simulink model "model_v4"  (R2023b)
settings: Solver=VariableStepAuto  StartTime=0.0  StopTime=10.0  RelTol=1e-3
(part 1 of 2)
settings Model: Creator=ian20030201  LastModifiedBy=ian20030201

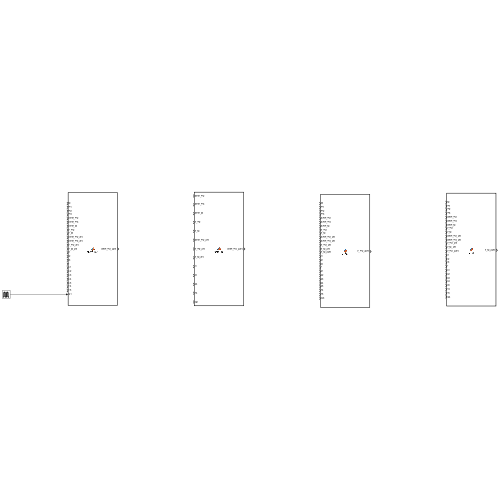
[thumbnail: Simulink's stored preview of the top-level diagram]
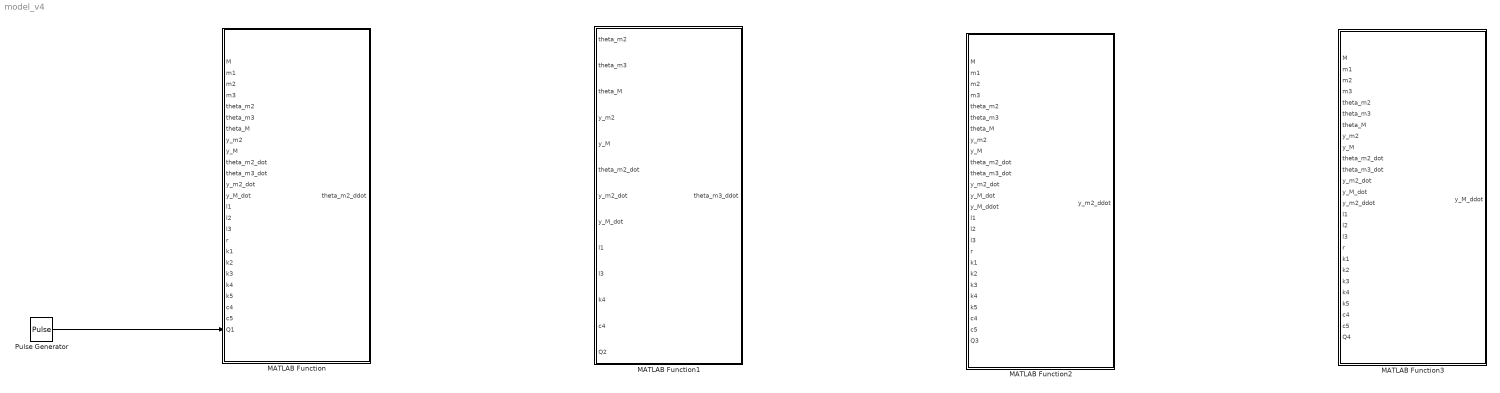
== system model_v4 ==
  MATLAB Function : MATLAB Function  TreatAsAtomicUnit=on
  MATLAB Function1 : MATLAB Function  TreatAsAtomicUnit=on
  MATLAB Function2 : MATLAB Function  TreatAsAtomicUnit=on
  MATLAB Function3 : MATLAB Function  TreatAsAtomicUnit=on
  Pulse Generator : DiscretePulseGenerator  PulseType=Time based  Period=10  PulseWidth=5
  wires:
  Pulse Generator/1 -> MATLAB Function/25(Q1)

== matlab function model_v4/MATLAB Function3 ==
  data: M input; y_M_ddot output; m1 input; m2 input; m3 input; theta_m2 input; theta_m3 input; theta_M input; y_m2 input; y_M input; theta_m2_dot input; theta_m3_dot input; y_m2_dot input; y_M_dot input; y_m2_ddot input; l1 input; l2 input; l3 input; r input; k1 input; k2 input; k3 input; k4 input; k5 input; c4 input; c5 input; Q4 input
function y_M_ddot = y_M(M, m1, m2, m3, theta_m2, theta_m3, theta_M, y_m2, y_M, theta_m2_dot, theta_m3_dot, y_m2_dot, y_M_dot, y_m2_ddot, l1, l2, l3, r, k1, k2, k3, k4, k5, c4, c5, Q4)

g = 9.81;
y_M_ddot = (-M*g*sqrt((l3*sin(theta_m3) - y_M*tan(theta_M) + y_m2*tan(theta_M))^2 + (l1*theta_m2 + l3*cos(theta_m3) - y_M - y_m2)^2)*(l3*sin(theta_m3) - y_M*tan(theta_M) + y_m2*tan(theta_M))^2*cos(theta_M)*tan(theta_M) - M*g*sqrt((l3*sin(theta_m3) - y_M*tan(theta_M) + y_m2*tan(theta_M))^2 + (l1*theta_m2 + l3*cos(theta_m3) - y_M - y_m2)^2)*(l1*theta_m2 + l3*cos(theta_m3) - y_M - y_m2)^2*cos(theta_M)*tan(theta_M) + Q4*sqrt((l3*sin(theta_m3) - y_M*tan(theta_M) + y_m2*tan(theta_M))^2 + (l1*theta_m2 + l3*cos(theta_m3) - y_M - y_m2)^2)*(l3*sin(theta_m3) - y_M*tan(theta_M) + y_m2*tan(theta_M))^2*tan(theta_M)^2 + Q4*sqrt((l3*sin(theta_m3) - y_M*tan(theta_M) + y_m2*tan(theta_M))^2 + (l1*theta_m2 + l3*cos(theta_m3) - y_M - y_m2)^2)*(l1*theta_m2 + l3*cos(theta_m3) - y_M - y_m2)^2*tan(theta_M)^2 + c4*l1^3*theta_m2^2*theta_m2_dot*sqrt((l3*sin(theta_m3) - y_M*tan(theta_M) + y_m2*tan(theta_M))^2 + (l1*theta_m2 + l3*cos(theta_m3) - y_M - y_m2)^2)*tan(theta_M)^2 - c4*l1^2*l3*theta_m2^2*theta_m3_dot*sqrt((l3*sin(theta_m3) - y_M*tan(theta_M) + y_m2*tan(theta_M))^2 + (l1*theta_m2 + l3*cos(theta_m3) - y_M - y_m2)^2)*sin(theta_m3)*tan(theta_M)^2 + c4*l1^2*l3*theta_m2*theta_m2_dot*sqrt((l3*sin(theta_m3) - y_M*tan(theta_M) + y_m2*tan(theta_M))^2 + (l1*theta_m2 + l3*cos(theta_m3) - y_M - y_m2)^2)*sin(theta_m3)*tan(theta_M)^3 + 2.0*c4*l1^2*l3*theta_m2*theta_m2_dot*sqrt((l3*sin(theta_m3) - y_M*tan(theta_M) + y_m2*tan(theta_M))^2 + (l1*theta_m2 + l3*cos(theta_m3) - y_M - y_m2)^2)*cos(theta_m3)*tan(theta_M)^2 - c4*l1^2*theta_m2^2*y_M_dot*sqrt((l3*sin(theta_m3) - y_M*tan(theta_M) + y_m2*tan(theta_M))^2 + (l1*theta_m2 + l3*cos(theta_m3) - y_M - y_m2)^2)*tan(theta_M)^2 - c4*l1^2*theta_m2^2*y_m2_dot*sqrt((l3*sin(theta_m3) - y_M*tan(theta_M) + y_m2*tan(theta_M))^2 + (l1*theta_m2 + l3*cos(theta_m3) - y_M - y_m2)^2)*tan(theta_M)^2 - c4*l1^2*theta_m2*theta_m2_dot*y_M*sqrt((l3*sin(theta_m3) - y_M*tan(theta_M) + y_m2*tan(theta_M))^2 + (l1*theta_m2 + l3*cos(theta_m3) - y_M - y_m2)^2)*tan(theta_M)^4 - 2.0*c4*l1^2*theta_m2*theta_m2_dot*y_M*sqrt((l3*sin(theta_m3) - y_M*tan(theta_M) + y_m2*tan(theta_M))^2 + (l1*theta_m2 + l3*cos(theta_m3) - y_M - y_m2)^2)*tan(theta_M)^2 + c4*l1^2*theta_m2*theta_m2_dot*y_m2*sqrt((l3*sin(theta_m3) - y_M*tan(theta_M) + y_m2*tan(theta_M))^2 + (l1*theta_m2 + l3*cos(theta_m3) - y_M - y_m2)^2)*tan(theta_M)^4 - 2.0*c4*l1^2*theta_m2*theta_m2_dot*y_m2*sqrt((l3*sin(theta_m3) - y_M*tan(theta_M) + y_m2*tan(theta_M))^2 + (l1*theta_m2 + l3*cos(theta_m3) - y_M - y_m2)^2)*tan(theta_M)^2 - c4*l1*l3^2*theta_m2*theta_m3_dot*sqrt((l3*sin(theta_m3) - y_M*tan(theta_M) + y_m2*tan(theta_M))^2 + (l1*theta_m2 + l3*cos(theta_m3) - y_M - y_m2)^2)*sin(theta_m3)^2*tan(theta_M)^3 - c4*l1*l3^2*theta_m2*theta_m3_dot*sqrt((l3*sin(theta_m3) - y_M*tan(theta_M) + y_m2*tan(theta_M))^2 + (l1*theta_m2 + l3*cos(theta_m3) - y_M - y_m2)^2)*sin(theta_m3)*cos(theta_m3)*tan(theta_M)^2 + c4*l1*l3^2*theta_m2_dot*sqrt((l3*sin(theta_m3) - y_M*tan(theta_M) + y_m2*tan(theta_M))^2 + (l1*theta_m2 + l3*cos(theta_m3) - y_M - y_m2)^2)*sin(theta_m3)*cos(theta_m3)*tan(theta_M)^3 + c4*l1*l3^2*theta_m2_dot*sqrt((l3*sin(theta_m3) - y_M*tan(theta_M) + y_m2*tan(theta_M))^2 + (l1*theta_m2 + l3*cos(theta_m3) - y_M - y_m2)^2)*cos(theta_m3)^2*tan(theta_M)^2 + c4*l1*l3*theta_m2*theta_m3_dot*y_M*sqrt((l3*sin(theta_m3) - y_M*tan(theta_M) + y_m2*tan(theta_M))^2 + (l1*theta_m2 + l3*cos(theta_m3) - y_M - y_m2)^2)*sin(theta_m3)*tan(theta_M)^4 + 2.0*c4*l1*l3*theta_m2*theta_m3_dot*y_M*sqrt((l3*sin(theta_m3) - y_M*tan(theta_M) + y_m2*tan(theta_M))^2 + (l1*theta_m2 + l3*cos(theta_m3) - y_M - y_m2)^2)*sin(theta_m3)*tan(theta_M)^2 - c4*l1*l3*theta_m2*theta_m3_dot*y_M*sqrt((l3*sin(theta_m3) - y_M*tan(theta_M) + y_m2*tan(theta_M))^2 + (l1*theta_m2 + l3*cos(theta_m3) - y_M - y_m2)^2)*cos(theta_m3)*tan(theta_M)^3 - c4*l1*l3*theta_m2*theta_m3_dot*y_m2*sqrt((l3*sin(theta_m3) - y_M*tan(theta_M) + y_m2*tan(theta_M))^2 + (l1*theta_m2 + l3*cos(theta_m3) - y_M - y_m2)^2)*sin(theta_m3)*tan(theta_M)^4 + 2.0*c4*l1*l3*theta_m2*theta_m3_dot*y_m2*sqrt((l3*sin(theta_m3) - y_M*tan(theta_M) + y_m2*tan(theta_M))^2 + (l1*theta_m2 + l3*cos(theta_m3) - y_M - y_m2)^2)*sin(theta_m3)*tan(theta_M)^2 + c4*l1*l3*theta_m2*theta_m3_dot*y_m2*sqrt((l3*sin(theta_m3) - y_M*tan(theta_M) + y_m2*tan(theta_M))^2 + (l1*theta_m2 + l3*cos(theta_m3) - y_M - y_m2)^2)*cos(theta_m3)*tan(theta_M)^3 - 2.0*c4*l1*l3*theta_m2*y_M_dot*sqrt((l3*sin(theta_m3) - y_M*tan(theta_M) + y_m2*tan(theta_M))^2 + (l1*theta_m2 + l3*cos(theta_m3) - y_M - y_m2)^2)*sin(theta_m3)*tan(theta_M)^3 - 2.0*c4*l1*l3*theta_m2*y_M_dot*sqrt((l3*sin(theta_m3) - y_M*tan(theta_M) + y_m2*tan(theta_M))^2 + (l1*theta_m2 + l3*cos(theta_m3) - y_M - y_m2)^2)*cos(theta_m3)*tan(theta_M)^2 - 2.0*c4*l1*l3*theta_m2*y_m2_dot*sqrt((l3*sin(theta_m3) - y_M*tan(theta_M) + y_m2*tan(theta_M))^2 + (l1*theta_m2 + l3*cos(theta_m3) - y_M - y_m2)^2)*cos(theta_m3)*tan(theta_M)^2 - c4*l1*l3*theta_m2_dot*y_M*sqrt((l3*sin(theta_m3) - y_M*tan(theta_M) + y_m2*tan(theta_M))^2 + (l1*theta_m2 + l3*cos(theta_m3) - y_M - y_m2)^2)*sin(theta_m3)*tan(theta_M)^3 - c4*l1*l3*theta_m2_dot*y_M*sqrt((l3*sin(theta_m3) - y_M*tan(theta_M) + y_m2*tan(theta_M))^2 + (l1*theta_m2 + l3*cos(theta_m3) - y_M - y_m2)^2)*cos(theta_m3)*tan(theta_M)^4 - 2.0*c4*l1*l3*theta_m2_dot*y_M*sqrt((l3*sin(theta_m3) - y_M*tan(theta_M) + y_m2*tan(theta_M))^2 + (l1*theta_m2 + l3*cos(theta_m3) - y_M - y_m2)^2)*cos(theta_m3)*tan(theta_M)^2 - c4*l1*l3*theta_m2_dot*y_m2*sqrt((l3*sin(theta_m3) - y_M*tan(theta_M) + y_m2*tan(theta_M))^2 + (l1*theta_m2 + l3*cos(theta_m3) - y_M - y_m2)^2)*sin(theta_m3)*tan(theta_M)^3 + c4*l1*l3*theta_m2_dot*y_m2*sqrt((l3*sin(theta_m3) - y_M*tan(theta_M) + y_m2*tan(theta_M))^2 + (l1*theta_m2 + l3*cos(theta_m3) - y_M - y_m2)^2)*cos(theta_m3)*tan(theta_M)^4 - 2.0*c4*l1*l3*theta_m2_dot*y_m2*sqrt((l3*sin(theta_m3) - y_M*tan(theta_M) + y_m2*tan(theta_M))^2 + (l1*theta_m2 + l3*cos(theta_m3) - y_M - y_m2)^2)*cos(theta_m3)*tan(theta_M)^2 + 2.0*c4*l1*theta_m2*y_M*y_M_dot*sqrt((l3*sin(theta_m3) - y_M*tan(theta_M) + y_m2*tan(theta_M))^2 + (l1*theta_m2 + l3*cos(theta_m3) - y_M - y_m2)^2)*tan(theta_M)^4 + 2.0*c4*l1*theta_m2*y_M*y_M_dot*sqrt((l3*sin(theta_m3) - y_M*tan(theta_M) + y_m2*tan(theta_M))^2 + (l1*theta_m2 + l3*cos(theta_m3) - y_M - y_m2)^2)*tan(theta_M)^2 + 2.0*c4*l1*theta_m2*y_M*y_m2_dot*sqrt((l3*sin(theta_m3) - y_M*tan(theta_M) + y_m2*tan(theta_M))^2 + (l1*theta_m2 + l3*cos(theta_m3) - y_M - y_m2)^2)*tan(theta_M)^2 - 2.0*c4*l1*theta_m2*y_M_dot*y_m2*sqrt((l3*sin(theta_m3) - y_M*tan(theta_M) + y_m2*tan(theta_M))^2 + (l1*theta_m2 + l3*cos(theta_m3) - y_M - y_m2)^2)*tan(theta_M)^4 + 2.0*c4*l1*theta_m2*y_M_dot*y_m2*sqrt((l3*sin(theta_m3) - y_M*tan(theta_M) + y_m2*tan(theta_M))^2 + (l1*theta_m2 + l3*cos(theta_m3) - y_M - y_m2)^2)*tan(theta_M)^2 + 2.0*c4*l1*theta_m2*y_m2*y_m2_dot*sqrt((l3*sin(theta_m3) - y_M*tan(theta_M) + y_m2*tan(theta_M))^2 + (l1*theta_m2 + l3*cos(theta_m3) - y_M - y_m2)^2)*tan(theta_M)^2 + c4*l1*theta_m2_dot*y_M^2*sqrt((l3*sin(theta_m3) - y_M*tan(theta_M) + y_m2*tan(theta_M))^2 + (l1*theta_m2 + l3*cos(theta_m3) - y_M - y_m2)^2)*tan(theta_M)^4 + c4*l1*theta_m2_dot*y_M^2*sqrt((l3*sin(theta_m3) - y_M*tan(theta_M) + y_m2*tan(theta_M))^2 + (l1*theta_m2 + l3*cos(theta_m3) - y_M - y_m2)^2)*tan(theta_M)^2 + 2.0*c4*l1*theta_m2_dot*y_M*y_m2*sqrt((l3*sin(theta_m3) - y_M*tan(theta_M) + y_m2*tan(theta_M))^2 + (l1*theta_m2 + l3*cos(theta_m3) - y_M - y_m2)^2)*tan(theta_M)^2 - c4*l1*theta_m2_dot*y_m2^2*sqrt((l3*sin(theta_m3) - y_M*tan(theta_M) + y_m2*tan(theta_M))^2 + (l1*theta_m2 + l3*cos(theta_m3) - y_M - y_m2)^2)*tan(theta_M)^4 + c4*l1*theta_m2_dot*y_m2^2*sqrt((l3*sin(theta_m3) - y_M*tan(theta_M) + y_m2*tan(theta_M))^2 + (l1*theta_m2 + l3*cos(theta_m3) - y_M - y_m2)^2)*tan(theta_M)^2 + c4*l3^2*theta_m3_dot*y_M*sqrt((l3*sin(theta_m3) - y_M*tan(theta_M) + y_m2*tan(theta_M))^2 + (l1*theta_m2 + l3*cos(theta_m3) - y_M - y_m2)^2)*sin(theta_m3)^2*tan(theta_M)^3 - c4*l3^2*theta_m3_dot*y_M*sqrt((l3*sin(theta_m3) - y_M*tan(theta_M) + y_m2*tan(theta_M))^2 + (l1*theta_m2 + l3*cos(theta_m3) - y_M - y_m2)^2)*sin(theta_m3)*cos(theta_m3)*tan(theta_M)^4 + c4*l3^2*theta_m3_dot*y_M*sqrt((l3*sin(theta_m3) - y_M*tan(theta_M) + y_m2*tan(theta_M))^2 + (l1*theta_m2 + l3*cos(theta_m3) - y_M - y_m2)^2)*sin(theta_m3)*cos(theta_m3)*tan(theta_M)^2 - c4*l3^2*theta_m3_dot*y_M*sqrt((l3*sin(theta_m3) - y_M*tan(theta_M) + y_m2*tan(theta_M))^2 + (l1*theta_m2 + l3*cos(theta_m3) - y_M - y_m2)^2)*cos(theta_m3)^2*tan(theta_M)^3 + c4*l3^2*theta_m3_dot*y_m2*sqrt((l3*sin(theta_m3) - y_M*tan(theta_M) + y_m2*tan(theta_M))^2 + (l1*theta_m2 + l3*cos(theta_m3) - y_M - y_m2)^2)*sin(theta_m3)^2*tan(theta_M)^3 + c4*l3^2*theta_m3_dot*y_m2*sqrt((l3*sin(theta_m3) - y_M*tan(theta_M) + y_m2*tan(theta_M))^2 + (l1*theta_m2 + l3*cos(theta_m3) - y_M - y_m2)^2)*sin(theta_m3)*cos(theta_m3)*tan(theta_M)^4 + c4*l3^2*theta_m3_dot*y_m2*sqrt((l3*sin(theta_m3) - y_M*tan(theta_M) + y_m2*tan(theta_M))^2 + (l1*theta_m2 + l3*cos(theta_m3) - y_M - y_m2)^2)*sin(theta_m3)*cos(theta_m3)*tan(theta_M)^2 + c4*l3^2*theta_m3_dot*y_m2*sqrt((l3*sin(theta_m3) - y_M*tan(theta_M) + y_m2*tan(theta_M))^2 + (l1*theta_m2 + l3*cos(theta_m3) - y_M - y_m2)^2)*cos(theta_m3)^2*tan(theta_M)^3 - c4*l3^2*y_M_dot*sqrt((l3*sin(theta_m3) - y_M*tan(theta_M) + y_m2*tan(theta_M))^2 + (l1*theta_m2 + l3*cos(theta_m3) - y_M - y_m2)^2)*sin(theta_m3)^2*tan(theta_M)^4 - 2.0*c4*l3^2*y_M_dot*sqrt((l3*sin(theta_m3) - y_M*tan(theta_M) + y_m2*tan(theta_M))^2 + (l1*theta_m2 + l3*cos(theta_m3) - y_M - y_m2)^2)*sin(theta_m3)*cos(theta_m3)*tan(theta_M)^3 - c4*l3^2*y_M_dot*sqrt((l3*sin(theta_m3) - y_M*tan(theta_M) + y_m2*tan(theta_M))^2 + (l1*theta_m2 + l3*cos(theta_m3) - y_M - y_m2)^2)*cos(theta_m3)^2*tan(theta_M)^2 + c4*l3^2*y_m2_dot*sqrt((l3*sin(theta_m3) - y_M*tan(theta_M) + y_m2*tan(theta_M))^2 + (l1*theta_m2 + l3*cos(theta_m3) - y_M - y_m2)^2)*sin(theta_m3)^2*tan(theta_M)^4 - c4*l3^2*y_m2_dot*sqrt((l3*sin(theta_m3) - y_M*tan(theta_M) + y_m2*tan(theta_M))^2 + (l1*theta_m2 + l3*cos(theta_m3) - y_M - y_m2)^2)*cos(theta_m3)^2*tan(theta_M)^2 - c4*l3*theta_m3_dot*y_M^2*sqrt((l3*sin(theta_m3) - y_M*tan(theta_M) + y_m2*tan(theta_M))^2 + (l1*theta_m2 + l3*cos(theta_m3) - y_M - y_m2)^2)*sin(theta_m3)*tan(theta_M)^4 - c4*l3*theta_m3_dot*y_M^2*sqrt((l3*sin(theta_m3) - y_M*tan(theta_M) + y_m2*tan(theta_M))^2 + (l1*theta_m2 + l3*cos(theta_m3) - y_M - y_m2)^2)*sin(theta_m3)*tan(theta_M)^2 + c4*l3*theta_m3_dot*y_M^2*sqrt((l3*sin(theta_m3) - y_M*tan(theta_M) + y_m2*tan(theta_M))^2 + (l1*theta_m2 + l3*cos(theta_m3) - y_M - y_m2)^2)*cos(theta_m3)*tan(theta_M)^5 + c4*l3*theta_m3_dot*y_M^2*sqrt((l3*sin(theta_m3) - y_M*tan(theta_M) + y_m2*tan(theta_M))^2 + (l1*theta_m2 + l3*cos(theta_m3) - y_M - y_m2)^2)*cos(theta_m3)*tan(theta_M)^3 - 2.0*c4*l3*theta_m3_dot*y_M*y_m2*sqrt((l3*sin(theta_m3) - y_M*tan(theta_M) + y_m2*tan(theta_M))^2 + (l1*theta_m2 + l3*cos(theta_m3) - y_M - y_m2)^2)*sin(theta_m3)*tan(theta_M)^2 - 2.0*c4*l3*theta_m3_dot*y_M*y_m2*sqrt((l3*sin(theta_m3) - y_M*tan(theta_M) + y_m2*tan(theta_M))^2 + (l1*theta_m2 + l3*cos(theta_m3) - y_M - y_m2)^2)*cos(theta_m3)*tan(theta_M)^5 + c4*l3*theta_m3_dot*y_m2^2*sqrt((l3*sin(theta_m3) - y_M*tan(theta_M) + y_m2*tan(theta_M))^2 + (l1*theta_m2 + l3*cos(theta_m3) - y_M - y_m2)^2)*sin(theta_m3)*tan(theta_M)^4 - c4*l3*theta_m3_dot*y_m2^2*sqrt((l3*sin(theta_m3) - y_M*tan(theta_M) + y_m2*tan(theta_M))^2 + (l1*theta_m2 + l3*cos(theta_m3) - y_M - y_m2)^2)*sin(theta_m3)*tan(theta_M)^2 + c4*l3*theta_m3_dot*y_m2^2*sqrt((l3*sin(theta_m3) - y_M*tan(theta_M) + y_m2*tan(theta_M))^2 + (l1*theta_m2 + l3*cos(theta_m3) - y_M - y_m2)^2)*cos(theta_m3)*tan(theta_M)^5 - c4*l3*theta_m3_dot*y_m2^2*sqrt((l3*sin(theta_m3) - y_M*tan(theta_M) + y_m2*tan(theta_M))^2 + (l1*theta_m2 + l3*cos(theta_m3) - y_M - y_m2)^2)*cos(theta_m3)*tan(theta_M)^3 + 2.0*c4*l3*y_M*y_M_dot*sqrt((l3*sin(theta_m3) - y_M*tan(theta_M) + y_m2*tan(theta_M))^2 + (l1*theta_m2 + l3*cos(theta_m3) - y_M - y_m2)^2)*sin(theta_m3)*tan(theta_M)^5 + 2.0*c4*l3*y_M*y_M_dot*sqrt((l3*sin(theta_m3) - y_M*tan(theta_M) + y_m2*tan(theta_M))^2 + (l1*theta_m2 + l3*cos(theta_m3) - y_M - y_m2)^2)*sin(theta_m3)*tan(theta_M)^3 + 2.0*c4*l3*y_M*y_M_dot*sqrt((l3*sin(theta_m3) - y_M*tan(theta_M) + y_m2*tan(theta_M))^2 + (l1*theta_m2 + l3*cos(theta_m3) - y_M - y_m2)^2)*cos(theta_m3)*tan(theta_M)^4 + 2.0*c4*l3*y_M*y_M_dot*sqrt((l3*sin(theta_m3) - y_M*tan(theta_M) + y_m2*tan(theta_M))^2 + (l1*theta_m2 + l3*cos(theta_m3) - y_M - y_m2)^2)*cos(theta_m3)*tan(theta_M)^2 - 2.0*c4*l3*y_M*y_m2_dot*sqrt((l3*sin(theta_m3) - y_M*tan(theta_M) + y_m2*tan(theta_M))^2 + (l1*theta_m2 + l3*cos(theta_m3) - y_M - y_m2)^2)*sin(theta_m3)*tan(theta_M)^5 + 2.0*c4*l3*y_M*y_m2_dot*sqrt((l3*sin(theta_m3) - y_M*tan(theta_M) + y_m2*tan(theta_M))^2 + (l1*theta_m2 + l3*cos(theta_m3) - y_M - y_m2)^2)*cos(theta_m3)*tan(theta_M)^2 - 2.0*c4*l3*y_M_dot*y_m2*sqrt((l3*sin(theta_m3) - y_M*tan(theta_M) + y_m2*tan(theta_M))^2 + (l1*theta_m2 + l3*cos(theta_m3) - y_M - y_m2)^2)*sin(theta_m3)*tan(theta_M)^5 + 2.0*c4*l3*y_M_dot*y_m2*sqrt((l3*sin(theta_m3) - y_M*tan(theta_M) + y_m2*tan(theta_M))^2 + (l1*theta_m2 + l3*cos(theta_m3) - y_M - y_m2)^2)*sin(theta_m3)*tan(theta_M)^3 - 2.0*c4*l3*y_M_dot*y_m2*sqrt((l3*sin(theta_m3) - y_M*tan(theta_M) + y_m2*tan(theta_M))^2 + (l1*theta_m2 + l3*cos(theta_m3) - y_M - y_m2)^2)*cos(theta_m3)*tan(theta_M)^4 + 2.0*c4*l3*y_M_dot*y_m2*sqrt((l3*sin(theta_m3) - y_M*tan(theta_M) + y_m2*tan(theta_M))^2 + (l1*theta_m2 + l3*cos(theta_m3) - y_M - y_m2)^2)*cos(theta_m3)*tan(theta_M)^2 + 2.0*c4*l3*y_m2*y_m2_dot*sqrt((l3*sin(theta_m3) - y_M*tan(theta_M) + y_m2*tan(theta_M))^2 + (l1*theta_m2 + l3*cos(theta_m3) - y_M - y_m2)^2)*sin(theta_m3)*tan(theta_M)^5 + 2.0*c4*l3*y_m2*y_m2_dot*sqrt((l3*sin(theta_m3) - y_M*tan(theta_M) + y_m2*tan(theta_M))^2 + (l1*theta_m2 + l3*cos(theta_m3) - y_M - y_m2)^2)*cos(theta_m3)*tan(theta_M)^2 - c4*y_M^2*y_M_dot*sqrt((l3*sin(theta_m3) - y_M*tan(theta_M) + y_m2*tan(theta_M))^2 + (l1*theta_m2 + l3*cos(theta_m3) - y_M - y_m2)^2)*tan(theta_M)^6 - 2.0*c4*y_M^2*y_M_dot*sqrt((l3*sin(theta_m3) - y_M*tan(theta_M) + y_m2*tan(theta_M))^2 + (l1*theta_m2 + l3*cos(theta_m3) - y_M - y_m2)^2)*tan(theta_M)^4 - c4*y_M^2*y_M_dot*sqrt((l3*sin(theta_m3) - y_M*tan(theta_M) + y_m2*tan(theta_M))^2 + (l1*theta_m2 + l3*cos(theta_m3) - y_M - y_m2)^2)*tan(theta_M)^2 + c4*y_M^2*y_m2_dot*sqrt((l3*sin(theta_m3) - y_M*tan(theta_M) + y_m2*tan(theta_M))^2 + (l1*theta_m2 + l3*cos(theta_m3) - y_M - y_m2)^2)*tan(theta_M)^6 - c4*y_M^2*y_m2_dot*sqrt((l3*sin(theta_m3) - y_M*tan(theta_M) + y_m2*tan(theta_M))^2 + (l1*theta_m2 + l3*cos(theta_m3) - y_M - y_m2)^2)*tan(theta_M)^2 + 2.0*c4*y_M*y_M_dot*y_m2*sqrt((l3*sin(theta_m3) - y_M*tan(theta_M) + y_m2*tan(theta_M))^2 + (l1*theta_m2 + l3*cos(theta_m3) - y_M - y_m2)^2)*tan(theta_M)^6 - 2.0*c4*y_M*y_M_dot*y_m2*sqrt((l3*sin(theta_m3) - y_M*tan(theta_M) + y_m2*tan(theta_M))^2 + (l1*theta_m2 + l3*cos(theta_m3) - y_M - y_m2)^2)*tan(theta_M)^2 - 2.0*c4*y_M*y_m2*y_m2_dot*sqrt((l3*sin(theta_m3) - y_M*tan(theta_M) + y_m2*tan(theta_M))^2 + (l1*theta_m2 + l3*cos(theta_m3) - y_M - y_m2)^2)*tan(theta_M)^6 - 2.0*c4*y_M*y_m2*y_m2_dot*sqrt((l3*sin(theta_m3) - y_M*tan(theta_M) + y_m2*tan(theta_M))^2 + (l1*theta_m2 + l3*cos(theta_m3) - y_M - y_m2)^2)*tan(theta_M)^2 - c4*y_M_dot*y_m2^2*sqrt((l3*sin(theta_m3) - y_M*tan(theta_M) + y_m2*tan(theta_M))^2 + (l1*theta_m2 + l3*cos(theta_m3) - y_M - y_m2)^2)*tan(theta_M)^6 + 2.0*c4*y_M_dot*y_m2^2*sqrt((l3*sin(theta_m3) - y_M*tan(theta_M) + y_m2*tan(theta_M))^2 + (l1*theta_m2 + l3*cos(theta_m3) - y_M - y_m2)^2)*tan(theta_M)^4 - c4*y_M_dot*y_m2^2*sqrt((l3*sin(theta_m3) - y_M*tan(theta_M) + y_m2*tan(theta_M))^2 + (l1*theta_m2 + l3*cos(theta_m3) - y_M - y_m2)^2)*tan(theta_M)^2 + c4*y_m2^2*y_m2_dot*sqrt((l3*sin(theta_m3) - y_M*tan(theta_M) + y_m2*tan(theta_M))^2 + (l1*theta_m2 + l3*cos(theta_m3) - y_M - y_m2)^2)*tan(theta_M)^6 - c4*y_m2^2*y_m2_dot*sqrt((l3*sin(theta_m3) - y_M*tan(theta_M) + y_m2*tan(theta_M))^2 + (l1*theta_m2 + l3*cos(theta_m3) - y_M - y_m2)^2)*tan(theta_M)^2 - c5*y_M_dot*sqrt((l3*sin(theta_m3) - y_M*tan(theta_M) + y_m2*tan(theta_M))^2 + (l1*theta_m2 + l3*cos(theta_m3) - y_M - y_m2)^2)*(l3*sin(theta_m3) - y_M*tan(theta_M) + y_m2*tan(theta_M))^2 - c5*y_M_dot*sqrt((l3*sin(theta_m3) - y_M*tan(theta_M) + y_m2*tan(theta_M))^2 + (l1*theta_m2 + l3*cos(theta_m3) - y_M - y_m2)^2)*(l1*theta_m2 + l3*cos(theta_m3) - y_M - y_m2)^2 + c5*y_m2_dot*sqrt((l3*sin(theta_m3) - y_M*tan(theta_M) + y_m2*tan(theta_M))^2 + (l1*theta_m2 + l3*cos(theta_m3) - y_M - y_m2)^2)*(l3*sin(theta_m3) - y_M*tan(theta_M) + y_m2*tan(theta_M))^2 + c5*y_m2_dot*sqrt((l3*sin(theta_m3) - y_M*tan(theta_M) + y_m2*tan(theta_M))^2 + (l1*theta_m2 + l3*cos(theta_m3) - y_M - y_m2)^2)*(l1*theta_m2 + l3*cos(theta_m3) - y_M - y_m2)^2 - k4*l1*l3*theta_m2*(l3*sin(theta_m3) - y_M*tan(theta_M) + y_m2*tan(theta_M))^2*tan(theta_M)^2 - k4*l1*l3*theta_m2*(l1*theta_m2 + l3*cos(theta_m3) - y_M - y_m2)^2*tan(theta_M)^2 + k4*l1*theta_m2*sqrt((l3*sin(theta_m3) - y_M*tan(theta_M) + y_m2*tan(theta_M))^2 + (l1*theta_m2 + l3*cos(theta_m3) - y_M - y_m2)^2)*(l3*sin(theta_m3) - y_M*tan(theta_M) + y_m2*tan(theta_M))^2*tan(theta_M)^2 + k4*l1*theta_m2*sqrt((l3*sin(theta_m3) - y_M*tan(theta_M) + y_m2*tan(theta_M))^2 + (l1*theta_m2 + l3*cos(theta_m3) - y_M - y_m2)^2)*(l1*theta_m2 + l3*cos(theta_m3) - y_M - y_m2)^2*tan(theta_M)^2 - k4*l3^2*(l3*sin(theta_m3) - y_M*tan(theta_M) + y_m2*tan(theta_M))^2*sin(theta_m3)*tan(theta_M)^3 - k4*l3^2*(l3*sin(theta_m3) - y_M*tan(theta_M) + y_m2*tan(theta_M))^2*cos(theta_m3)*tan(theta_M)^2 - k4*l3^2*(l1*theta_m2 + l3*cos(theta_m3) - y_M - y_m2)^2*sin(theta_m3)*tan(theta_M)^3 - k4*l3^2*(l1*theta_m2 + l3*cos(theta_m3) - y_M - y_m2)^2*cos(theta_m3)*tan(theta_M)^2 + k4*l3*y_M*(l3*sin(theta_m3) - y_M*tan(theta_M) + y_m2*tan(theta_M))^2*tan(theta_M)^4 + k4*l3*y_M*(l3*sin(theta_m3) - y_M*tan(theta_M) + y_m2*tan(theta_M))^2*tan(theta_M)^2 + k4*l3*y_M*(l1*theta_m2 + l3*cos(theta_m3) - y_M - y_m2)^2*tan(theta_M)^4 + k4*l3*y_M*(l1*theta_m2 + l3*cos(theta_m3) - y_M - y_m2)^2*tan(theta_M)^2 - k4*l3*y_m2*(l3*sin(theta_m3) - y_M*tan(theta_M) + y_m2*tan(theta_M))^2*tan(theta_M)^4 + k4*l3*y_m2*(l3*sin(theta_m3) - y_M*tan(theta_M) + y_m2*tan(theta_M))^2*tan(theta_M)^2 - k4*l3*y_m2*(l1*theta_m2 + l3*cos(theta_m3) - y_M - y_m2)^2*tan(theta_M)^4 + k4*l3*y_m2*(l1*theta_m2 + l3*cos(theta_m3) - y_M - y_m2)^2*tan(theta_M)^2 + k4*l3*sqrt((l3*sin(theta_m3) - y_M*tan(theta_M) + y_m2*tan(theta_M))^2 + (l1*theta_m2 + l3*cos(theta_m3) - y_M - y_m2)^2)*(l3*sin(theta_m3) - y_M*tan(theta_M) + y_m2*tan(theta_M))^2*sin(theta_m3)*tan(theta_M)^3 + k4*l3*sqrt((l3*sin(theta_m3) - y_M*tan(theta_M) + y_m2*tan(theta_M))^2 + (l1*theta_m2 + l3*cos(theta_m3) - y_M - y_m2)^2)*(l3*sin(theta_m3) - y_M*tan(theta_M) + y_m2*tan(theta_M))^2*cos(theta_m3)*tan(theta_M)^2 + k4*l3*sqrt((l3*sin(theta_m3) - y_M*tan(theta_M) + y_m2*tan(theta_M))^2 + (l1*theta_m2 + l3*cos(theta_m3) - y_M - y_m2)^2)*(l1*theta_m2 + l3*cos(theta_m3) - y_M - y_m2)^2*sin(theta_m3)*tan(theta_M)^3 + k4*l3*sqrt((l3*sin(theta_m3) - y_M*tan(theta_M) + y_m2*tan(theta_M))^2 + (l1*theta_m2 + l3*cos(theta_m3) - y_M - y_m2)^2)*(l1*theta_m2 + l3*cos(theta_m3) - y_M - y_m2)^2*cos(theta_m3)*tan(theta_M)^2 - k4*y_M*sqrt((l3*sin(theta_m3) - y_M*tan(theta_M) + y_m2*tan(theta_M))^2 + (l1*theta_m2 + l3*cos(theta_m3) - y_M - y_m2)^2)*(l3*sin(theta_m3) - y_M*tan(theta_M) + y_m2*tan(theta_M))^2*tan(theta_M)^4 - k4*y_M*sqrt((l3*sin(theta_m3) - y_M*tan(theta_M) + y_m2*tan(theta_M))^2 + (l1*theta_m2 + l3*cos(theta_m3) - y_M - y_m2)^2)*(l3*sin(theta_m3) - y_M*tan(theta_M) + y_m2*tan(theta_M))^2*tan(theta_M)^2 - k4*y_M*sqrt((l3*sin(theta_m3) - y_M*tan(theta_M) + y_m2*tan(theta_M))^2 + (l1*theta_m2 + l3*cos(theta_m3) - y_M - y_m2)^2)*(l1*theta_m2 + l3*cos(theta_m3) - y_M - y_m2)^2*tan(theta_M)^4 - k4*y_M*sqrt((l3*sin(theta_m3) - y_M*tan(theta_M) + y_m2*tan(theta_M))^2 + (l1*theta_m2 + l3*cos(theta_m3) - y_M - y_m2)^2)*(l1*theta_m2 + l3*cos(theta_m3) - y_M - y_m2)^2*tan(theta_M)^2 + k4*y_m2*sqrt((l3*sin(theta_m3) - y_M*tan(theta_M) + y_m2*tan(theta_M))^2 + (l1*theta_m2 + l3*cos(theta_m3) - y_M - y_m2)^2)*(l3*sin(theta_m3) - y_M*tan(theta_M) + y_m2*tan(theta_M))^2*tan(theta_M)^4 - k4*y_m2*sqrt((l3*sin(theta_m3) - y_M*tan(theta_M) + y_m2*tan(theta_M))^2 + (l1*theta_m2 + l3*cos(theta_m3) - y_M - y_m2)^2)*(l3*sin(theta_m3) - y_M*tan(theta_M) + y_m2*tan(theta_M))^2*tan(theta_M)^2 + k4*y_m2*sqrt((l3*sin(theta_m3) - y_M*tan(theta_M) + y_m2*tan(theta_M))^2 + (l1*theta_m2 + l3*cos(theta_m3) - y_M - y_m2)^2)*(l1*theta_m2 + l3*cos(theta_m3) - y_M - y_m2)^2*tan(theta_M)^4 - k4*y_m2*sqrt((l3*sin(theta_m3) - y_M*tan(theta_M) + y_m2*tan(theta_M))^2 + (l1*theta_m2 + l3*cos(theta_m3) - y_M - y_m2)^2)*(l1*theta_m2 + l3*cos(theta_m3) - y_M - y_m2)^2*tan(theta_M)^2 - k5*y_M*sqrt((l3*sin(theta_m3) - y_M*tan(theta_M) + y_m2*tan(theta_M))^2 + (l1*theta_m2 + l3*cos(theta_m3) - y_M - y_m2)^2)*(l3*sin(theta_m3) - y_M*tan(theta_M) + y_m2*tan(theta_M))^2 - k5*y_M*sqrt((l3*sin(theta_m3) - y_M*tan(theta_M) + y_m2*tan(theta_M))^2 + (l1*theta_m2 + l3*cos(theta_m3) - y_M - y_m2)^2)*(l1*theta_m2 + l3*cos(theta_m3) - y_M - y_m2)^2 + k5*y_m2*sqrt((l3*sin(theta_m3) - y_M*tan(theta_M) + y_m2*tan(theta_M))^2 + (l1*theta_m2 + l3*cos(theta_m3) - y_M - y_m2)^2)*(l3*sin(theta_m3) - y_M*tan(theta_M) + y_m2*tan(theta_M))^2 + k5*y_m2*sqrt((l3*sin(theta_m3) - y_M*tan(theta_M) + y_m2*tan(theta_M))^2 + (l1*theta_m2 + l3*cos(theta_m3) - y_M - y_m2)^2)*(l1*theta_m2 + l3*cos(theta_m3) - y_M - y_m2)^2 + m1*y_m2_ddot*sqrt((l3*sin(theta_m3) - y_M*tan(theta_M) + y_m2*tan(theta_M))^2 + (l1*theta_m2 + l3*cos(theta_m3) - y_M - y_m2)^2)*(l3*sin(theta_m3) - y_M*tan(theta_M) + y_m2*tan(theta_M))^2*tan(theta_M)^4 + m1*y_m2_ddot*sqrt((l3*sin(theta_m3) - y_M*tan(theta_M) + y_m2*tan(theta_M))^2 + (l1*theta_m2 + l3*cos(theta_m3) - y_M - y_m2)^2)*(l1*theta_m2 + l3*cos(theta_m3) - y_M - y_m2)^2*tan(theta_M)^4 + m2*y_m2_ddot*sqrt((l3*sin(theta_m3) - y_M*tan(theta_M) + y_m2*tan(theta_M))^2 + (l1*theta_m2 + l3*cos(theta_m3) - y_M - y_m2)^2)*(l3*sin(theta_m3) - y_M*tan(theta_M) + y_m2*tan(theta_M))^2*tan(theta_M)^4 + m2*y_m2_ddot*sqrt((l3*sin(theta_m3) - y_M*tan(theta_M) + y_m2*tan(theta_M))^2 + (l1*theta_m2 + l3*cos(theta_m3) - y_M - y_m2)^2)*(l1*theta_m2 + l3*cos(theta_m3) - y_M - y_m2)^2*tan(theta_M)^4 + m3*y_m2_ddot*sqrt((l3*sin(theta_m3) - y_M*tan(theta_M) + y_m2*tan(theta_M))^2 + (l1*theta_m2 + l3*cos(theta_m3) - y_M - y_m2)^2)*(l3*sin(theta_m3) - y_M*tan(theta_M) + y_m2*tan(theta_M))^2*tan(theta_M)^4 + m3*y_m2_ddot*sqrt((l3*sin(theta_m3) - y_M*tan(theta_M) + y_m2*tan(theta_M))^2 + (l1*theta_m2 + l3*cos(theta_m3) - y_M - y_m2)^2)*(l1*theta_m2 + l3*cos(theta_m3) - y_M - y_m2)^2*tan(theta_M)^4)/(sqrt((l3*sin(theta_m3) - y_M*tan(theta_M) + y_m2*tan(theta_M))^2 + (l1*theta_m2 + l3*cos(theta_m3) - y_M - y_m2)^2)*(M*(l3*sin(theta_m3) - y_M*tan(theta_M) + y_m2*tan(theta_M))^2 + M*(l1*theta_m2 + l3*cos(theta_m3) - y_M - y_m2)^2 + m1*(l3*sin(theta_m3) - y_M*tan(theta_M) + y_m2*tan(theta_M))^2*tan(theta_M)^2 + m1*(l1*theta_m2 + l3*cos(theta_m3) - y_M - y_m2)^2*tan(theta_M)^2 + m2*(l3*sin(theta_m3) - y_M*tan(theta_M) + y_m2*tan(theta_M))^2*tan(theta_M)^2 + m2*(l1*theta_m2 + l3*cos(theta_m3) - y_M - y_m2)^2*tan(theta_M)^2 + m3*(l3*sin(theta_m3) - y_M*tan(theta_M) + y_m2*tan(theta_M))^2*tan(theta_M)^2 + m3*(l1*theta_m2 + l3*cos(theta_m3) - y_M - y_m2)^2*tan(theta_M)^2)*tan(theta_M)^2);

== matlab function model_v4/MATLAB Function1 ==
  data: theta_m2 input; theta_m3 input; theta_M input; y_m2 input; y_M input; theta_m2_dot input; y_m2_dot input; y_M_dot input; l1 input; l3 input; k4 input; c4 input; Q2 input; theta_m3_ddot output
function theta_m3_ddot = theta_m3(theta_m2, theta_m3, theta_M, y_m2, y_M, theta_m2_dot, y_m2_dot, y_M_dot, l1, l3, k4, c4, Q2)

theta_m3_ddot = (-c4*l3*sqrt((l3*sin(theta_m3) - y_M*tan(theta_M) + y_m2*tan(theta_M))^2 + (l1*theta_m2 + l3*cos(theta_m3) - y_M - y_m2)^2)*(-l1^3*theta_m2^2*theta_m2_dot*sin(theta_m3) - 0.5*l1^2*l3*theta_m2*theta_m2_dot*sin(2.0*theta_m3) + l1^2*theta_m2^2*y_M_dot*sin(theta_m3) + l1^2*theta_m2^2*y_m2_dot*sin(theta_m3) + 2.0*l1^2*theta_m2*theta_m2_dot*y_M*sin(theta_m3) - l1^2*theta_m2*theta_m2_dot*y_M*cos(theta_m3)*tan(theta_M) + 2.0*l1^2*theta_m2*theta_m2_dot*y_m2*sin(theta_m3) + l1^2*theta_m2*theta_m2_dot*y_m2*cos(theta_m3)*tan(theta_M) + 0.5*l1*l3*theta_m2*y_M_dot*sin(2.0*theta_m3) - 0.5*l1*l3*theta_m2*y_M_dot*cos(2.0*theta_m3)*tan(theta_M) + 0.5*l1*l3*theta_m2*y_M_dot*tan(theta_M) + 0.5*l1*l3*theta_m2*y_m2_dot*sin(2.0*theta_m3) + 0.5*l1*l3*theta_m2*y_m2_dot*cos(2.0*theta_m3)*tan(theta_M) - 0.5*l1*l3*theta_m2*y_m2_dot*tan(theta_M) + 0.5*l1*l3*theta_m2_dot*y_M*sin(2.0*theta_m3) - 0.5*l1*l3*theta_m2_dot*y_M*cos(2.0*theta_m3)*tan(theta_M) - 0.5*l1*l3*theta_m2_dot*y_M*tan(theta_M) + 0.5*l1*l3*theta_m2_dot*y_m2*sin(2.0*theta_m3) + 0.5*l1*l3*theta_m2_dot*y_m2*cos(2.0*theta_m3)*tan(theta_M) + 0.5*l1*l3*theta_m2_dot*y_m2*tan(theta_M) - l1*theta_m2*y_M*y_M_dot*sin(theta_m3)*tan(theta_M)^2 - 2.0*l1*theta_m2*y_M*y_M_dot*sin(theta_m3) + l1*theta_m2*y_M*y_M_dot*cos(theta_m3)*tan(theta_M) + l1*theta_m2*y_M*y_m2_dot*sin(theta_m3)*tan(theta_M)^2 - 2.0*l1*theta_m2*y_M*y_m2_dot*sin(theta_m3) + l1*theta_m2*y_M*y_m2_dot*cos(theta_m3)*tan(theta_M) + l1*theta_m2*y_M_dot*y_m2*sin(theta_m3)*tan(theta_M)^2 - 2.0*l1*theta_m2*y_M_dot*y_m2*sin(theta_m3) - l1*theta_m2*y_M_dot*y_m2*cos(theta_m3)*tan(theta_M) - l1*theta_m2*y_m2*y_m2_dot*sin(theta_m3)*tan(theta_M)^2 - 2.0*l1*theta_m2*y_m2*y_m2_dot*sin(theta_m3) - l1*theta_m2*y_m2*y_m2_dot*cos(theta_m3)*tan(theta_M) - l1*theta_m2_dot*y_M^2*sin(theta_m3) + l1*theta_m2_dot*y_M^2*cos(theta_m3)*tan(theta_M) - 2.0*l1*theta_m2_dot*y_M*y_m2*sin(theta_m3) - l1*theta_m2_dot*y_m2^2*sin(theta_m3) - l1*theta_m2_dot*y_m2^2*cos(theta_m3)*tan(theta_M) + 0.5*l3*y_M*y_M_dot*sin(2.0*theta_m3)*tan(theta_M)^2 - 0.5*l3*y_M*y_M_dot*sin(2.0*theta_m3) + l3*y_M*y_M_dot*cos(2.0*theta_m3)*tan(theta_M) - 0.5*l3*y_M*y_m2_dot*sin(2.0*theta_m3)*tan(theta_M)^2 - 0.5*l3*y_M*y_m2_dot*sin(2.0*theta_m3) + l3*y_M*y_m2_dot*tan(theta_M) - 0.5*l3*y_M_dot*y_m2*sin(2.0*theta_m3)*tan(theta_M)^2 - 0.5*l3*y_M_dot*y_m2*sin(2.0*theta_m3) - l3*y_M_dot*y_m2*tan(theta_M) + 0.5*l3*y_m2*y_m2_dot*sin(2.0*theta_m3)*tan(theta_M)^2 - 0.5*l3*y_m2*y_m2_dot*sin(2.0*theta_m3) - l3*y_m2*y_m2_dot*cos(2.0*theta_m3)*tan(theta_M) + y_M^2*y_M_dot*sin(theta_m3)*tan(theta_M)^2 + y_M^2*y_M_dot*sin(theta_m3) - y_M^2*y_M_dot*cos(theta_m3)*tan(theta_M)^3 - y_M^2*y_M_dot*cos(theta_m3)*tan(theta_M) - y_M^2*y_m2_dot*sin(theta_m3)*tan(theta_M)^2 + y_M^2*y_m2_dot*sin(theta_m3) + y_M^2*y_m2_dot*cos(theta_m3)*tan(theta_M)^3 - y_M^2*y_m2_dot*cos(theta_m3)*tan(theta_M) + 2.0*y_M*y_M_dot*y_m2*sin(theta_m3) + 2.0*y_M*y_M_dot*y_m2*cos(theta_m3)*tan(theta_M)^3 + 2.0*y_M*y_m2*y_m2_dot*sin(theta_m3) - 2.0*y_M*y_m2*y_m2_dot*cos(theta_m3)*tan(theta_M)^3 - y_M_dot*y_m2^2*sin(theta_m3)*tan(theta_M)^2 + y_M_dot*y_m2^2*sin(theta_m3) - y_M_dot*y_m2^2*cos(theta_m3)*tan(theta_M)^3 + y_M_dot*y_m2^2*cos(theta_m3)*tan(theta_M) + y_m2^2*y_m2_dot*sin(theta_m3)*tan(theta_M)^2 + y_m2^2*y_m2_dot*sin(theta_m3) + y_m2^2*y_m2_dot*cos(theta_m3)*tan(theta_M)^3 + y_m2^2*y_m2_dot*cos(theta_m3)*tan(theta_M)) + k4*l3^2*(-l1*theta_m2*(l3*sin(theta_m3) - y_M*tan(theta_M) + y_m2*tan(theta_M))^2*sin(theta_m3) - l1*theta_m2*(l1*theta_m2 + l3*cos(theta_m3) - y_M - y_m2)^2*sin(theta_m3) + y_M*(l3*sin(theta_m3) - y_M*tan(theta_M) + y_m2*tan(theta_M))^2*sin(theta_m3) - y_M*(l3*sin(theta_m3) - y_M*tan(theta_M) + y_m2*tan(theta_M))^2*cos(theta_m3)*tan(theta_M) + y_M*(l1*theta_m2 + l3*cos(theta_m3) - y_M - y_m2)^2*sin(theta_m3) - y_M*(l1*theta_m2 + l3*cos(theta_m3) - y_M - y_m2)^2*cos(theta_m3)*tan(theta_M) + y_m2*(l3*sin(theta_m3) - y_M*tan(theta_M) + y_m2*tan(theta_M))^2*sin(theta_m3) + y_m2*(l3*sin(theta_m3) - y_M*tan(theta_M) + y_m2*tan(theta_M))^2*cos(theta_m3)*tan(theta_M) + y_m2*(l1*theta_m2 + l3*cos(theta_m3) - y_M - y_m2)^2*sin(theta_m3) + y_m2*(l1*theta_m2 + l3*cos(theta_m3) - y_M - y_m2)^2*cos(theta_m3)*tan(theta_M)) + 8.0*((0.25*y_M^2 - 0.5*y_M*y_m2 + 0.25*y_m2^2 + (0.25*l1^2*theta_m2^2 + 0.5*l1*l3*theta_m2*cos(theta_m3) - 0.5*l1*theta_m2*y_M - 0.5*l1*theta_m2*y_m2 + 0.25*l3^2 - 0.5*l3*y_M*sin(theta_m3)*tan(theta_M) - 0.5*l3*y_M*cos(theta_m3) + 0.5*l3*y_m2*sin(theta_m3)*tan(theta_M) - 0.5*l3*y_m2*cos(theta_m3) + y_M*y_m2)*cos(theta_M)^2)/cos(theta_M)^2)^(3/2)*(Q2 + k4*l1*l3*theta_m2*sin(theta_m3) - k4*l3*y_M*sin(theta_m3) + k4*l3*y_M*cos(theta_m3)*tan(theta_M) - k4*l3*y_m2*sin(theta_m3) - k4*l3*y_m2*cos(theta_m3)*tan(theta_M)))/(c4*l3^2*sqrt((l3*sin(theta_m3) - y_M*tan(theta_M) + y_m2*tan(theta_M))^2 + (l1*theta_m2 + l3*cos(theta_m3) - y_M - y_m2)^2)*(-l1*theta_m2*sin(theta_m3) + y_M*sin(theta_m3) - y_M*cos(theta_m3)*tan(theta_M) + y_m2*sin(theta_m3) + y_m2*cos(theta_m3)*tan(theta_M))^2);

== matlab function model_v4/MATLAB Function ==
  data: M input; theta_m2_ddot output; m1 input; m2 input; m3 input; theta_m2 input; theta_m3 input; theta_M input; y_m2 input; y_M input; theta_m2_dot input; theta_m3_dot input; y_m2_dot input; y_M_dot input; l1 input; l2 input; l3 input; r input; k1 input; k2 input; k3 input; k4 input; k5 input; c4 input; c5 input; Q1 input
function theta_m2_ddot = theta_m2(M, m1, m2, m3, theta_m2, theta_m3, theta_M, y_m2, y_M, theta_m2_dot, theta_m3_dot, y_m2_dot, y_M_dot, l1, l2, l3, r, k1, k2, k3, k4, k5, c4, c5, Q1)

g = 9.81;
theta_m2_ddot = (Q1*y_M^2 - 2.0*Q1*y_M*y_m2 + Q1*y_m2^2 - c4*l1^2*theta_m2*y_M*y_M_dot + c4*l1^2*theta_m2*y_M*y_m2_dot + c4*l1^2*theta_m2*y_M_dot*y_m2 - c4*l1^2*theta_m2*y_m2*y_m2_dot - c4*l1*l3*y_M*y_M_dot*cos(theta_m3) + c4*l1*l3*y_M*y_m2_dot*cos(theta_m3) + c4*l1*l3*y_M_dot*y_m2*cos(theta_m3) - c4*l1*l3*y_m2*y_m2_dot*cos(theta_m3) + c4*l1*y_M^2*y_M_dot - c4*l1*y_M^2*y_m2_dot - c4*l1*y_M_dot*y_m2^2 + c4*l1*y_m2^2*y_m2_dot - g*l1*m1*y_M^2*cos(theta_m2) + 2.0*g*l1*m1*y_M*y_m2*cos(theta_m2) - g*l1*m1*y_m2^2*cos(theta_m2) + g*l1*m3*y_M^2*cos(theta_m2) - 2.0*g*l1*m3*y_M*y_m2*cos(theta_m2) + g*l1*m3*y_m2^2*cos(theta_m2) - 0.5*k1*l1^2*y_M^2*sin(2.0*theta_m2) + k1*l1^2*y_M*y_m2*sin(2.0*theta_m2) - 0.5*k1*l1^2*y_m2^2*sin(2.0*theta_m2) - k1*l1*y_M^2*y_m2*cos(theta_m2) + 2.0*k1*l1*y_M*y_m2^2*cos(theta_m2) - k1*l1*y_m2^3*cos(theta_m2) - 0.5*k3*l1^2*y_M^2*sin(2.0*theta_m2) + k3*l1^2*y_M*y_m2*sin(2.0*theta_m2) - 0.5*k3*l1^2*y_m2^2*sin(2.0*theta_m2) + k3*l1*y_M^2*y_m2*cos(theta_m2) - 2.0*k3*l1*y_M*y_m2^2*cos(theta_m2) + k3*l1*y_m2^3*cos(theta_m2) - k4*l1^2*theta_m2*y_M^2 + 2.0*k4*l1^2*theta_m2*y_M*y_m2 - k4*l1^2*theta_m2*y_m2^2 - k4*l1*l3*y_M^2*cos(theta_m3) + 2.0*k4*l1*l3*y_M*y_m2*cos(theta_m3) - k4*l1*l3*y_m2^2*cos(theta_m3) + k4*l1*y_M^3 - k4*l1*y_M^2*y_m2 - k4*l1*y_M*y_m2^2 + k4*l1*y_m2^3 + (Q1*l1^2*theta_m2^2 + 2.0*Q1*l1*l3*theta_m2*cos(theta_m3) - 2.0*Q1*l1*theta_m2*y_M - 2.0*Q1*l1*theta_m2*y_m2 + Q1*l3^2 - 2.0*Q1*l3*y_M*sin(theta_m3)*tan(theta_M) - 2.0*Q1*l3*y_M*cos(theta_m3) + 2.0*Q1*l3*y_m2*sin(theta_m3)*tan(theta_M) - 2.0*Q1*l3*y_m2*cos(theta_m3) + 4.0*Q1*y_M*y_m2 - c4*l1^4*theta_m2^2*theta_m2_dot + c4*l1^3*l3*theta_m2^2*theta_m3_dot*sin(theta_m3) - 2.0*c4*l1^3*l3*theta_m2*theta_m2_dot*cos(theta_m3) + c4*l1^3*theta_m2^2*y_M_dot + c4*l1^3*theta_m2^2*y_m2_dot + 2.0*c4*l1^3*theta_m2*theta_m2_dot*y_M + 2.0*c4*l1^3*theta_m2*theta_m2_dot*y_m2 + 0.5*c4*l1^2*l3^2*theta_m2*theta_m3_dot*sin(2.0*theta_m3) - 0.5*c4*l1^2*l3^2*theta_m2_dot*cos(2.0*theta_m3) - 0.5*c4*l1^2*l3^2*theta_m2_dot - 2.0*c4*l1^2*l3*theta_m2*theta_m3_dot*y_M*sin(theta_m3) + c4*l1^2*l3*theta_m2*theta_m3_dot*y_M*cos(theta_m3)*tan(theta_M) - 2.0*c4*l1^2*l3*theta_m2*theta_m3_dot*y_m2*sin(theta_m3) - c4*l1^2*l3*theta_m2*theta_m3_dot*y_m2*cos(theta_m3)*tan(theta_M) + c4*l1^2*l3*theta_m2*y_M_dot*sin(theta_m3)*tan(theta_M) + 2.0*c4*l1^2*l3*theta_m2*y_M_dot*cos(theta_m3) - c4*l1^2*l3*theta_m2*y_m2_dot*sin(theta_m3)*tan(theta_M) + 2.0*c4*l1^2*l3*theta_m2*y_m2_dot*cos(theta_m3) + 2.0*c4*l1^2*l3*theta_m2_dot*y_M*cos(theta_m3) + 2.0*c4*l1^2*l3*theta_m2_dot*y_m2*cos(theta_m3) - c4*l1^2*theta_m2*y_M*y_M_dot - 3.0*c4*l1^2*theta_m2*y_M*y_m2_dot - 3.0*c4*l1^2*theta_m2*y_M_dot*y_m2 - c4*l1^2*theta_m2*y_m2*y_m2_dot - c4*l1^2*theta_m2_dot*y_M^2 - 2.0*c4*l1^2*theta_m2_dot*y_M*y_m2 - c4*l1^2*theta_m2_dot*y_m2^2 - 0.5*c4*l1*l3^2*theta_m3_dot*y_M*sin(2.0*theta_m3) + 0.5*c4*l1*l3^2*theta_m3_dot*y_M*cos(2.0*theta_m3)*tan(theta_M) + 0.5*c4*l1*l3^2*theta_m3_dot*y_M*tan(theta_M) - 0.5*c4*l1*l3^2*theta_m3_dot*y_m2*sin(2.0*theta_m3) - 0.5*c4*l1*l3^2*theta_m3_dot*y_m2*cos(2.0*theta_m3)*tan(theta_M) - 0.5*c4*l1*l3^2*theta_m3_dot*y_m2*tan(theta_M) + 0.5*c4*l1*l3^2*y_M_dot*sin(2.0*theta_m3)*tan(theta_M) + 0.5*c4*l1*l3^2*y_M_dot*cos(2.0*theta_m3) + 0.5*c4*l1*l3^2*y_M_dot - 0.5*c4*l1*l3^2*y_m2_dot*sin(2.0*theta_m3)*tan(theta_M) + 0.5*c4*l1*l3^2*y_m2_dot*cos(2.0*theta_m3) + 0.5*c4*l1*l3^2*y_m2_dot + c4*l1*l3*theta_m3_dot*y_M^2*sin(theta_m3) - c4*l1*l3*theta_m3_dot*y_M^2*cos(theta_m3)*tan(theta_M) + 2.0*c4*l1*l3*theta_m3_dot*y_M*y_m2*sin(theta_m3) + c4*l1*l3*theta_m3_dot*y_m2^2*sin(theta_m3) + c4*l1*l3*theta_m3_dot*y_m2^2*cos(theta_m3)*tan(theta_M) - c4*l1*l3*y_M*y_M_dot*sin(theta_m3)*tan(theta_M) - c4*l1*l3*y_M*y_M_dot*cos(theta_m3) + c4*l1*l3*y_M*y_m2_dot*sin(theta_m3)*tan(theta_M) - 3.0*c4*l1*l3*y_M*y_m2_dot*cos(theta_m3) - c4*l1*l3*y_M_dot*y_m2*sin(theta_m3)*tan(theta_M) - 3.0*c4*l1*l3*y_M_dot*y_m2*cos(theta_m3) + c4*l1*l3*y_m2*y_m2_dot*sin(theta_m3)*tan(theta_M) - c4*l1*l3*y_m2*y_m2_dot*cos(theta_m3) + 2.0*c4*l1*y_M^2*y_m2_dot + 2.0*c4*l1*y_M*y_M_dot*y_m2 + 2.0*c4*l1*y_M*y_m2*y_m2_dot + 2.0*c4*l1*y_M_dot*y_m2^2 - g*l1^3*m1*theta_m2^2*cos(theta_m2) + g*l1^3*m3*theta_m2^2*cos(theta_m2) - g*l1^2*l3*m1*theta_m2*cos(theta_m2 - theta_m3) - g*l1^2*l3*m1*theta_m2*cos(theta_m2 + theta_m3) + g*l1^2*l3*m3*theta_m2*cos(theta_m2 - theta_m3) + g*l1^2*l3*m3*theta_m2*cos(theta_m2 + theta_m3) + 2.0*g*l1^2*m1*theta_m2*y_M*cos(theta_m2) + 2.0*g*l1^2*m1*theta_m2*y_m2*cos(theta_m2) - 2.0*g*l1^2*m3*theta_m2*y_M*cos(theta_m2) - 2.0*g*l1^2*m3*theta_m2*y_m2*cos(theta_m2) - g*l1*l3^2*m1*cos(theta_m2) + g*l1*l3^2*m3*cos(theta_m2) - g*l1*l3*m1*y_M*sin(theta_m2 - theta_m3)*tan(theta_M) + g*l1*l3*m1*y_M*sin(theta_m2 + theta_m3)*tan(theta_M) + g*l1*l3*m1*y_M*cos(theta_m2 - theta_m3) + g*l1*l3*m1*y_M*cos(theta_m2 + theta_m3) + g*l1*l3*m1*y_m2*sin(theta_m2 - theta_m3)*tan(theta_M) - g*l1*l3*m1*y_m2*sin(theta_m2 + theta_m3)*tan(theta_M) + g*l1*l3*m1*y_m2*cos(theta_m2 - theta_m3) + g*l1*l3*m1*y_m2*cos(theta_m2 + theta_m3) + g*l1*l3*m3*y_M*sin(theta_m2 - theta_m3)*tan(theta_M) - g*l1*l3*m3*y_M*sin(theta_m2 + theta_m3)*tan(theta_M) - g*l1*l3*m3*y_M*cos(theta_m2 - theta_m3) - g*l1*l3*m3*y_M*cos(theta_m2 + theta_m3) - g*l1*l3*m3*y_m2*sin(theta_m2 - theta_m3)*tan(theta_M) + g*l1*l3*m3*y_m2*sin(theta_m2 + theta_m3)*tan(theta_M) - g*l1*l3*m3*y_m2*cos(theta_m2 - theta_m3) - g*l1*l3*m3*y_m2*cos(theta_m2 + theta_m3) - 4.0*g*l1*m1*y_M*y_m2*cos(theta_m2) + 4.0*g*l1*m3*y_M*y_m2*cos(theta_m2) - 0.5*k1*l1^4*theta_m2^2*sin(2.0*theta_m2) - 0.5*k1*l1^3*l3*theta_m2*sin(2.0*theta_m2 - theta_m3) - 0.5*k1*l1^3*l3*theta_m2*sin(2.0*theta_m2 + theta_m3) - k1*l1^3*theta_m2^2*y_m2*cos(theta_m2) + k1*l1^3*theta_m2*y_M*sin(2.0*theta_m2) + k1*l1^3*theta_m2*y_m2*sin(2.0*theta_m2) - 0.5*k1*l1^2*l3^2*sin(2.0*theta_m2) - k1*l1^2*l3*theta_m2*y_m2*cos(theta_m2 - theta_m3) - k1*l1^2*l3*theta_m2*y_m2*cos(theta_m2 + theta_m3) + 0.5*k1*l1^2*l3*y_M*sin(2.0*theta_m2 - theta_m3) + 0.5*k1*l1^2*l3*y_M*sin(2.0*theta_m2 + theta_m3) + 0.5*k1*l1^2*l3*y_M*cos(2.0*theta_m2 - theta_m3)*tan(theta_M) - 0.5*k1*l1^2*l3*y_M*cos(2.0*theta_m2 + theta_m3)*tan(theta_M) + 0.5*k1*l1^2*l3*y_m2*sin(2.0*theta_m2 - theta_m3) + 0.5*k1*l1^2*l3*y_m2*sin(2.0*theta_m2 + theta_m3) - 0.5*k1*l1^2*l3*y_m2*cos(2.0*theta_m2 - theta_m3)*tan(theta_M) + 0.5*k1*l1^2*l3*y_m2*cos(2.0*theta_m2 + theta_m3)*tan(theta_M) + 2.0*k1*l1^2*theta_m2*y_M*y_m2*cos(theta_m2) + 2.0*k1*l1^2*theta_m2*y_m2^2*cos(theta_m2) - 2.0*k1*l1^2*y_M*y_m2*sin(2.0*theta_m2) - k1*l1*l3^2*y_m2*cos(theta_m2) - k1*l1*l3*y_M*y_m2*sin(theta_m2 - theta_m3)*tan(theta_M) + k1*l1*l3*y_M*y_m2*sin(theta_m2 + theta_m3)*tan(theta_M) + k1*l1*l3*y_M*y_m2*cos(theta_m2 - theta_m3) + k1*l1*l3*y_M*y_m2*cos(theta_m2 + theta_m3) + k1*l1*l3*y_m2^2*sin(theta_m2 - theta_m3)*tan(theta_M) - k1*l1*l3*y_m2^2*sin(theta_m2 + theta_m3)*tan(theta_M) + k1*l1*l3*y_m2^2*cos(theta_m2 - theta_m3) + k1*l1*l3*y_m2^2*cos(theta_m2 + theta_m3) - 4.0*k1*l1*y_M*y_m2^2*cos(theta_m2) - 0.5*k3*l1^4*theta_m2^2*sin(2.0*theta_m2) - 0.5*k3*l1^3*l3*theta_m2*sin(2.0*theta_m2 - theta_m3) - 0.5*k3*l1^3*l3*theta_m2*sin(2.0*theta_m2 + theta_m3) + k3*l1^3*theta_m2^2*y_m2*cos(theta_m2) + k3*l1^3*theta_m2*y_M*sin(2.0*theta_m2) + k3*l1^3*theta_m2*y_m2*sin(2.0*theta_m2) - 0.5*k3*l1^2*l3^2*sin(2.0*theta_m2) + k3*l1^2*l3*theta_m2*y_m2*cos(theta_m2 - theta_m3) + k3*l1^2*l3*theta_m2*y_m2*cos(theta_m2 + theta_m3) + 0.5*k3*l1^2*l3*y_M*sin(2.0*theta_m2 - theta_m3) + 0.5*k3*l1^2*l3*y_M*sin(2.0*theta_m2 + theta_m3) + 0.5*k3*l1^2*l3*y_M*cos(2.0*theta_m2 - theta_m3)*tan(theta_M) - 0.5*k3*l1^2*l3*y_M*cos(2.0*theta_m2 + theta_m3)*tan(theta_M) + 0.5*k3*l1^2*l3*y_m2*sin(2.0*theta_m2 - theta_m3) + 0.5*k3*l1^2*l3*y_m2*sin(2.0*theta_m2 + theta_m3) - 0.5*k3*l1^2*l3*y_m2*cos(2.0*theta_m2 - theta_m3)*tan(theta_M) + 0.5*k3*l1^2*l3*y_m2*cos(2.0*theta_m2 + theta_m3)*tan(theta_M) - 2.0*k3*l1^2*theta_m2*y_M*y_m2*cos(theta_m2) - 2.0*k3*l1^2*theta_m2*y_m2^2*cos(theta_m2) - 2.0*k3*l1^2*y_M*y_m2*sin(2.0*theta_m2) + k3*l1*l3^2*y_m2*cos(theta_m2) + k3*l1*l3*y_M*y_m2*sin(theta_m2 - theta_m3)*tan(theta_M) - k3*l1*l3*y_M*y_m2*sin(theta_m2 + theta_m3)*tan(theta_M) - k3*l1*l3*y_M*y_m2*cos(theta_m2 - theta_m3) - k3*l1*l3*y_M*y_m2*cos(theta_m2 + theta_m3) - k3*l1*l3*y_m2^2*sin(theta_m2 - theta_m3)*tan(theta_M) + k3*l1*l3*y_m2^2*sin(theta_m2 + theta_m3)*tan(theta_M) - k3*l1*l3*y_m2^2*cos(theta_m2 - theta_m3) - k3*l1*l3*y_m2^2*cos(theta_m2 + theta_m3) + 4.0*k3*l1*y_M*y_m2^2*cos(theta_m2) - k4*l1^4*theta_m2^3 - 3.0*k4*l1^3*l3*theta_m2^2*cos(theta_m3) + 3.0*k4*l1^3*theta_m2^2*y_M + 3.0*k4*l1^3*theta_m2^2*y_m2 - k4*l1^2*l3^2*theta_m2*cos(2.0*theta_m3) - 2.0*k4*l1^2*l3^2*theta_m2 + 2.0*k4*l1^2*l3*theta_m2*y_M*sin(theta_m3)*tan(theta_M) + 6.0*k4*l1^2*l3*theta_m2*y_M*cos(theta_m3) - 2.0*k4*l1^2*l3*theta_m2*y_m2*sin(theta_m3)*tan(theta_M) + 6.0*k4*l1^2*l3*theta_m2*y_m2*cos(theta_m3) + 2.0*k4*l1^2*l3*theta_m2*sqrt((0.5*y_M^2 - y_M*y_m2 + 0.5*y_m2^2 + (cos(2.0*theta_M) + 1.0)*(0.25*l1^2*theta_m2^2 + 0.5*l1*l3*theta_m2*cos(theta_m3) - 0.5*l1*theta_m2*y_M - 0.5*l1*theta_m2*y_m2 + 0.25*l3^2 - 0.5*l3*y_M*sin(theta_m3)*tan(theta_M) - 0.5*l3*y_M*cos(theta_m3) + 0.5*l3*y_m2*sin(theta_m3)*tan(theta_M) - 0.5*l3*y_m2*cos(theta_m3) + y_M*y_m2))/(cos(2.0*theta_M) + 1.0)) - 2.0*k4*l1^2*theta_m2*y_M^2 - 8.0*k4*l1^2*theta_m2*y_M*y_m2 - 2.0*k4*l1^2*theta_m2*y_m2^2 - k4*l1*l3^3*cos(theta_m3) + k4*l1*l3^2*y_M*sin(2.0*theta_m3)*tan(theta_M) + k4*l1*l3^2*y_M*cos(2.0*theta_m3) + 2.0*k4*l1*l3^2*y_M - k4*l1*l3^2*y_m2*sin(2.0*theta_m3)*tan(theta_M) + k4*l1*l3^2*y_m2*cos(2.0*theta_m3) + 2.0*k4*l1*l3^2*y_m2 + 2.0*k4*l1*l3^2*sqrt((0.5*y_M^2 - y_M*y_m2 + 0.5*y_m2^2 + (cos(2.0*theta_M) + 1.0)*(0.25*l1^2*theta_m2^2 + 0.5*l1*l3*theta_m2*cos(theta_m3) - 0.5*l1*theta_m2*y_M - 0.5*l1*theta_m2*y_m2 + 0.25*l3^2 - 0.5*l3*y_M*sin(theta_m3)*tan(theta_M) - 0.5*l3*y_M*cos(theta_m3) + 0.5*l3*y_m2*sin(theta_m3)*tan(theta_M) - 0.5*l3*y_m2*cos(theta_m3) + y_M*y_m2))/(cos(2.0*theta_M) + 1.0))*cos(theta_m3) - 2.0*k4*l1*l3*y_M^2*sin(theta_m3)*tan(theta_M) - 2.0*k4*l1*l3*y_M^2*cos(theta_m3) - 8.0*k4*l1*l3*y_M*y_m2*cos(theta_m3) - 2.0*k4*l1*l3*y_M*sqrt((0.5*y_M^2 - y_M*y_m2 + 0.5*y_m2^2 + (cos(2.0*theta_M) + 1.0)*(0.25*l1^2*theta_m2^2 + 0.5*l1*l3*theta_m2*cos(theta_m3) - 0.5*l1*theta_m2*y_M - 0.5*l1*theta_m2*y_m2 + 0.25*l3^2 - 0.5*l3*y_M*sin(theta_m3)*tan(theta_M) - 0.5*l3*y_M*cos(theta_m3) + 0.5*l3*y_m2*sin(theta_m3)*tan(theta_M) - 0.5*l3*y_m2*cos(theta_m3) + y_M*y_m2))/(cos(2.0*theta_M) + 1.0)) + 2.0*k4*l1*l3*y_m2^2*sin(theta_m3)*tan(theta_M) - 2.0*k4*l1*l3*y_m2^2*cos(theta_m3) - 2.0*k4*l1*l3*y_m2*sqrt((0.5*y_M^2 - y_M*y_m2 + 0.5*y_m2^2 + (cos(2.0*theta_M) + 1.0)*(0.25*l1^2*theta_m2^2 + 0.5*l1*l3*theta_m2*cos(theta_m3) - 0.5*l1*theta_m2*y_M - 0.5*l1*theta_m2*y_m2 + 0.25*l3^2 - 0.5*l3*y_M*sin(theta_m3)*tan(theta_M) - 0.5*l3*y_M*cos(theta_m3) + 0.5*l3*y_m2*sin(theta_m3)*tan(theta_M) - 0.5*l3*y_m2*cos(theta_m3) + y_M*y_m2))/(cos(2.0*theta_M) + 1.0)) + 4.0*k4*l1*y_M^2*y_m2 + 4.0*k4*l1*y_M*y_m2^2)*cos(theta_M)^2)/(l1^2*(m1*y_M^2 - 2.0*m1*y_M*y_m2 + m1*y_m2^2 + m3*y_M^2 - 2.0*m3*y_M*y_m2 + m3*y_m2^2 + (l1^2*m1*theta_m2^2 + l1^2*m3*theta_m2^2 + 2.0*l1*l3*m1*theta_m2*cos(theta_m3) + 2.0*l1*l3*m3*theta_m2*cos(theta_m3) - 2.0*l1*m1*theta_m2*y_M - 2.0*l1*m1*theta_m2*y_m2 - 2.0*l1*m3*theta_m2*y_M - 2.0*l1*m3*theta_m2*y_m2 + l3^2*m1 + l3^2*m3 - 2.0*l3*m1*y_M*sin(theta_m3)*tan(theta_M) - 2.0*l3*m1*y_M*cos(theta_m3) + 2.0*l3*m1*y_m2*sin(theta_m3)*tan(theta_M) - 2.0*l3*m1*y_m2*cos(theta_m3) - 2.0*l3*m3*y_M*sin(theta_m3)*tan(theta_M) - 2.0*l3*m3*y_M*cos(theta_m3) + 2.0*l3*m3*y_m2*sin(theta_m3)*tan(theta_M) - 2.0*l3*m3*y_m2*cos(theta_m3) + 4.0*m1*y_M*y_m2 + 4.0*m3*y_M*y_m2)*cos(theta_M)^2));
